simulink model "MS_QD2_QBP_manual_R2023"  (R2023a)
settings: Solver=ode2  StartTime=0.0  StopTime=inf  FixedStep=0.001  RelTol=1e-3  EnableMultiTasking=on
undefined symbols (not defined in the file): qc_get_step_size
libraries: quarc_library x61, simulink x8, simulink_extras x1
(part 2 of 2)

== system MS_QD2_QBP_manual_R2023/MISSION SERVER LEADER FOLLOWER CONTROL/Subsystem5/Triggered Subsystem4 ==
  Time (s) : Inport
  Trigger : TriggerPort  VariantControl=(inherit)
  Print2 : quarc_library/User Interface/Standard I//O/Print  format_string=[ %lf ] (s): JOYSTICK ISSUE \n  max_code_units=512  optimization=Minimizing latency  sample_time=-1  active=off
      settings: SourceProductName=QUARC Targets
  Terminator : Terminator
  Terminator1 : Terminator
  wires:
  Print2/1 -> Terminator1/1
  Print2/2 -> Terminator/1
  Time (s)/1 -> Print2/1

== system MS_QD2_QBP_manual_R2023/MISSION SERVER LEADER FOLLOWER CONTROL/Subsystem5/Triggered Subsystem5 ==
  Time (s) : Inport
  Trigger : TriggerPort  VariantControl=(inherit)
  Print2 : quarc_library/User Interface/Standard I//O/Print  format_string=[ %lf ] (s): START FOLLOWING \n  max_code_units=512  optimization=Minimizing latency  sample_time=-1  active=off
      settings: SourceProductName=QUARC Targets
  Terminator : Terminator
  Terminator1 : Terminator
  wires:
  Time (s)/1 -> Print2/1
  Print2/2 -> Terminator/1
  Print2/1 -> Terminator1/1

== system MS_QD2_QBP_manual_R2023/MISSION SERVER LEADER FOLLOWER CONTROL/Subsystem5/Triggered Subsystem6 ==
  Time (s) : Inport
  Trigger : TriggerPort  TriggerType=falling  VariantControl=(inherit)
  Print2 : quarc_library/User Interface/Standard I//O/Print  format_string=[ %lf ] (s): STOP FOLLOWING \n  max_code_units=512  optimization=Minimizing latency  sample_time=-1  active=off
      settings: SourceProductName=QUARC Targets
  Terminator : Terminator
  Terminator1 : Terminator
  wires:
  Time (s)/1 -> Print2/1
  Print2/2 -> Terminator/1
  Print2/1 -> Terminator1/1

== system MS_QD2_QBP_manual_R2023/MISSION SERVER LEADER FOLLOWER CONTROL/Subsystem5/Triggered Subsystem7 ==
  Time (s) : Inport
  Trigger : TriggerPort  TriggerType=falling  VariantControl=(inherit)
  Print2 : quarc_library/User Interface/Standard I//O/Print  format_string=[ %lf ] (s): DRONE LANDING \n  max_code_units=512  optimization=Minimizing latency  sample_time=-1  active=off
      settings: SourceProductName=QUARC Targets
  Terminator : Terminator
  Terminator1 : Terminator
  wires:
  Time (s)/1 -> Print2/1
  Print2/1 -> Terminator1/1
  Print2/2 -> Terminator/1

== system MS_QD2_QBP_manual_R2023/MISSION SERVER LEADER FOLLOWER CONTROL/StopAllSignal/Subsystem/Triggered Subsystem1 ==
  Trigger : TriggerPort  VariantControl=(inherit)
  Print : quarc_library/User Interface/Standard I//O/Print  format_string="Communication with QDrone Stopped, stopping all models  \\n"  max_code_units=512  optimization=Minimizing latency  sample_time=-1  active=off
      settings: SourceProductName=QUARC Targets

== system MS_QD2_QBP_manual_R2023/MISSION SERVER LEADER FOLLOWER CONTROL/StopAllSignal/Subsystem/Triggered Subsystem2 ==
  Trigger : TriggerPort  VariantControl=(inherit)
  Constant : Constant
  StopAllModels : Outport  InitialOutput=[0]
  wires:
  Constant/1 -> StopAllModels/1

== system MS_QD2_QBP_manual_R2023/MISSION SERVER LEADER FOLLOWER CONTROL/StopAllSignal/Subsystem1/Triggered Subsystem1 ==
  Trigger : TriggerPort  VariantControl=(inherit)
  Print : quarc_library/User Interface/Standard I//O/Print  format_string="Joystick triggers not back - Place them away from you and run again  \\n"  max_code_units=512  optimization=Minimizing latency  sample_time=-1  active=off
      settings: SourceProductName=QUARC Targets

== system MS_QD2_QBP_manual_R2023/MISSION SERVER LEADER FOLLOWER CONTROL/StopAllSignal/Subsystem1/Triggered Subsystem2 ==
  Trigger : TriggerPort  VariantControl=(inherit)
  Constant : Constant
  StopAllModels : Outport  InitialOutput=[0]
  wires:
  Constant/1 -> StopAllModels/1

== system MS_QD2_QBP_manual_R2023/MISSION SERVER LEADER FOLLOWER CONTROL/StopAllSignal/Subsystem2/Triggered Subsystem1 ==
  Trigger : TriggerPort  VariantControl=(inherit)
  Print : quarc_library/User Interface/Standard I//O/Print  format_string="Not tracking on start - Make sure correct vehicles are used  \\n"  max_code_units=512  optimization=Minimizing latency  sample_time=-1  active=off
      settings: SourceProductName=QUARC Targets

== system MS_QD2_QBP_manual_R2023/MISSION SERVER LEADER FOLLOWER CONTROL/StopAllSignal/Subsystem2/Triggered Subsystem2 ==
  Trigger : TriggerPort  VariantControl=(inherit)
  Constant : Constant
  StopAllModels : Outport  InitialOutput=[0]
  wires:
  Constant/1 -> StopAllModels/1

== system MS_QD2_QBP_manual_R2023/MISSION SERVER LEADER FOLLOWER CONTROL/StopAllSignal/Subsystem3/Triggered Subsystem1 ==
  Trigger : TriggerPort  VariantControl=(inherit)
  Print : quarc_library/User Interface/Standard I//O/Print  format_string="Emergency stop pressed  \\n"  max_code_units=512  optimization=Minimizing latency  sample_time=-1  active=off
      settings: SourceProductName=QUARC Targets

== system MS_QD2_QBP_manual_R2023/MISSION SERVER LEADER FOLLOWER CONTROL/StopAllSignal/Subsystem3/Triggered Subsystem2 ==
  Trigger : TriggerPort  VariantControl=(inherit)
  Constant : Constant
  StopAllModels : Outport  InitialOutput=[0]
  wires:
  Constant/1 -> StopAllModels/1

== system MS_QD2_QBP_manual_R2023/MISSION SERVER LEADER FOLLOWER CONTROL/StopAllSignal/Subsystem4/Triggered Subsystem1 ==
  Trigger : TriggerPort  VariantControl=(inherit)
  Print : quarc_library/User Interface/Standard I//O/Print  format_string="Stopped due to drone landing  \\n"  max_code_units=512  optimization=Minimizing latency  sample_time=-1  active=off
      settings: SourceProductName=QUARC Targets

== system MS_QD2_QBP_manual_R2023/MISSION SERVER LEADER FOLLOWER CONTROL/StopAllSignal/Subsystem4/Triggered Subsystem2 ==
  Trigger : TriggerPort  VariantControl=(inherit)
  Constant : Constant
  StopAllModels : Outport  InitialOutput=[0]
  wires:
  Constant/1 -> StopAllModels/1

== system MS_QD2_QBP_manual_R2023/MISSION SERVER LEADER FOLLOWER CONTROL/StopAllSignal/Subsystem4/Triggered Subsystem3 ==
  Trigger : TriggerPort  TriggerType=falling  VariantControl=(inherit)
  Constant : Constant
  Autoland Triggered : Outport  InitialOutput=[0]
  wires:
  Constant/1 -> Autoland Triggered/1

== system MS_QD2_QBP_manual_R2023/MISSION SERVER LEADER FOLLOWER CONTROL/StopAllSignal/Subsystem5/Triggered Subsystem1 ==
  Trigger : TriggerPort  VariantControl=(inherit)
  Print : quarc_library/User Interface/Standard I//O/Print  format_string=One of the vehicles not placed correctly. Camera should look at back wall. \n  max_code_units=512  optimization=Minimizing latency  sample_time=-1  active=off
      settings: SourceProductName=QUARC Targets

== system MS_QD2_QBP_manual_R2023/MISSION SERVER LEADER FOLLOWER CONTROL/StopAllSignal/Subsystem5/Triggered Subsystem2 ==
  Trigger : TriggerPort  VariantControl=(inherit)
  Constant : Constant
  StopAllModels : Outport  InitialOutput=[0]
  wires:
  Constant/1 -> StopAllModels/1

== matlab function MS_QD2_QBP_manual_R2023/MISSION SERVER LEADER FOLLOWER CONTROL/QBotData/Extract Object Data ==
  data: data input; position output; orientation output; index input; tracking output
function [position, orientation, tracking] = fcn(data, index)

n = length(data)/7;

if (index<=0)||(index>n)
    position = zeros(1,3); orientation = zeros(1,3); tracking = 0;
else
    position = [data(index*7 -6) data(index*7 -5) data(index*7 -4)];
    orientation = [data(index*7 -3) data(index*7 -2) data(index*7 -1)];
    tracking = data(index*7);
end

== matlab function MS_QD2_QBP_manual_R2023/MISSION SERVER LEADER FOLLOWER CONTROL/QDroneData/Extract Object Data ==
  data: data input; position output; orientation output; index input; tracking output

function [position, orientation, tracking] = fcn(data, index)

n = length(data)/7;


% position = data((index-1)*3 + 1: (index-1)*3 + 3);
% orientation = data( 3*n + 3*(index-1) + 1: 3*n + 3*(index-1) + 3);
% tracking = data(end-n+index - 1);


if (index<=0)||(index>n)
    position = zeros(1,3); orientation = zeros(1,3); tracking = 0;
else
    position = [data(index*7 -6) data(index*7 -5) data(index*7 -4)];
    orientation = [data(index*7 -3) data(index*7 -2) data(index*7 -1)];
    tracking = data(index*7);
end

== matlab function MS_QD2_QBP_manual_R2023/Communication/Detect Communication loss/MATLAB Function ==
  data: time input; stream_connection_loss output; state input; error input
function stream_connection_loss  = fcn(time, state, error)

stream_connection_loss = 0;
if time > 1
    if ~((state == 2)&&(error >= 0))
        % stream connection is not established correctly
        stream_connection_loss = 1;
    end
end
